simulink library "DQN_Lib (conflicted copy 2023-11-25 155310)"  (R2023b)
settings: Solver=VariableStepAuto  StartTime=0.0  StopTime=10.0  RelTol=1e-3
undefined symbols (not defined in the file): FreqRad, HrmOrd, Init, La, N, R, Ra, TimeStep, Ts, Ts_dqn, Ws
libraries: $bdroot x4, spsMeanVariableFrequencyLib x4, eeTransforms x3, spsabctodq0Lib x2, spsAlphaBetaZerotodq0Lib x1
(part 5 of 8)

== matlab function DQN_Lib (conflicted copy 2023-11-25 155310)/DQn->ABC11 ==
  data: Xdc input size=3; Xdp input; Xdn input; Xdz input; Xqp input; Xqn input; Xqz input; th input; abc output; N parameter
%function abc = Mult(Z0,Zdp,Zqp,Zdn,Zqn,Zdz,Zqz,th, N)
function abc = dqn2abc(Xdc,Xdp,Xdn,Xdz,Xqp,Xqn,Xqz,th,N)



abc   = [Xdc(1);Xdc(2);Xdc(3)];
abc3p = [0;0;0];
abc3n = [0;0;0];
abc1p = [0;0;0];
%abc1n = [0;0;0];
   

for i = 1 : N
    abc3p = abc3p + [sin(i*th)*Xdp(i)           + cos(i*th)*Xqp(i);
                     sin(i*th-2*pi/3)*Xdp(i)    + cos(i*th-2*pi/3)*Xqp(i);
                     sin(i*th+2*pi/3)*Xdp(i)    + cos(i*th+2*pi/3)*Xqp(i)];
                 
    abc3n = abc3n + [sin(-i*th)*Xdn(i)          + cos(-i*th)*Xqn(i);
                     sin(-i*th-2*pi/3)*Xdn(i)   + cos(-i*th-2*pi/3)*Xqn(i);
                     sin(-i*th+2*pi/3)*Xdn(i)   + cos(-i*th+2*pi/3)*Xqn(i)];
                 
    abc1p = abc1p + [sin(i*th)*Xdz(i)           + cos(i*th)*Xqz(i);
                     sin(i*th-0*2*pi/3)*Xdz(i)  + cos(i*th-0*2*pi/3)*Xqz(i);
                     sin(i*th+0*2*pi/3)*Xdz(i)  + cos(i*th+0*2*pi/3)*Xqz(i)];  
 
%     abc1n = abc1n + [sin(-i*th)*D1n(i)           + cos(-i*th)*Q1n(i);
%                      sin(-i*th-0*2*pi/3)*D1n(i)  + cos(-i*th-0*2*pi/3)*Q1n(i);
%                      sin(-i*th+0*2*pi/3)*D1n(i)  + cos(-i*th+0*2*pi/3)*Q1n(i)];  
                 
end

abc = abc+abc3p+abc3n+abc1p;%+abc1n;

== matlab function DQN_Lib (conflicted copy 2023-11-25 155310)/MATLAB Function ==
  data: Xdp input; X_DQN output; Xdn input; Xdz input; Xqp input; Xqn input; Xqz input; N parameter
function X_DQN = fcn(Xdp, Xdn, Xdz, Xqp, Xqn, Xqz, N)

    X_DQN = zeros(N+1,6);

    X_DQN(:,1) = Xdp;
    X_DQN(:,2) = Xdn;
    X_DQN(:,3) = Xdz;
    X_DQN(:,4) = Xqp;
    X_DQN(:,5) = Xqn;
    X_DQN(:,6) = Xqz;

end

== matlab function DQN_Lib (conflicted copy 2023-11-25 155310)/Int_DQN_fdbk/Int_d_2N_2 ==
  settings: updateMethod=DISCRETE
  data: Zdp output; Xdp input; Xdn input; Xdz input; Xqp input; Xqn input; Xqz input; Zdn output; N parameter; dt parameter; w parameter; Zdz output; Zqp output; Zqn output; Zqz output; R parameter; iL parameter; SW parameter
function [Zdp,Zdn,Zdz,Zqp,Zqn,Zqz]  = IntDQN(Xdp, Xdn, Xdz, Xqp, Xqn, Xqz, N, dt, w, R, iL, SW)

    persistent Zdc_old;    
    persistent Xdc_old;   
    persistent Zdp_old;    
    persistent Zqp_old;    
    persistent Zdn_old;    
    persistent Zqn_old;    
    persistent Zdz_old;    
    persistent Zqz_old;  
    persistent Krl1;
    persistent Krl2;
       
    persistent dt2;
    persistent range;
       
    Xdc = zeros(6,1);
    Zdc = zeros(6,1);
    
    Xdc(1) = Xdp(1);
    Xdc(2) = Xdn(1);
    Xdc(3) = Xdz(1);
    Xdc(4) = Xqp(1);
    Xdc(5) = Xqn(1);
    Xdc(6) = Xqz(1);

    Xdp = [Xdp(2:end); zeros(N-numel(Xdp)+1,1)];
    Xqp = [Xqp(2:end); zeros(N-numel(Xqp)+1,1)];
    Xdn = [Xdn(2:end); zeros(N-numel(Xdn)+1,1)];
    Xqn = [Xqn(2:end); zeros(N-numel(Xqn)+1,1)];
    Xdz = [Xdz(2:end); zeros(N-numel(Xdz)+1,1)];
    Xqz = [Xqz(2:end); zeros(N-numel(Xqz)+1,1)];
       
    Zdp = zeros(N+1,1);
    Zdn = zeros(N+1,1);
    Zqp = zeros(N+1,1);
    Zqn = zeros(N+1,1);
    Zdz = zeros(N+1,1);
    Zqz = zeros(N+1,1);
       
    if(isempty(Zdp_old)) 
        Zdc_old  = zeros(6,1); %Zdc_old  = InitInt';
        Xdc_old  = zeros(6,1);
        
        Zdp_old  = zeros(N,1);% Zdp_old(1) = InitInt(1);
        Zdn_old  = zeros(N,1);% Zdn_old(1) = InitInt(2);
        Zdz_old  = zeros(N,1);% Zdz_old(1) = InitInt(3);
        Zqp_old  = zeros(N,1);% Zqp_old(1) = InitInt(4);
        Zqn_old  = zeros(N,1);% Zqn_old(1) = InitInt(5);
        Zqz_old  = zeros(N,1);% Zqz_old(1) = InitInt(6);
        
        dt2 = dt/2;  
        range = N; 
        
        if(SW)
            Krl1 = (iL/(1+dt2*R*iL));
            Krl2 = (1-dt2*R*iL)/(1+dt2*R*iL);
        else
            Krl1 = 1;
            Krl2 = 1;
        end
        
    end

    
    
    %Zdc(:) = dt2*(Xdc(:)+Xdc_old(:))+Zdc_old(:);
    Zdc(:) = Krl1*dt2*(Xdc(:)+Xdc_old(:))+Krl2*Zdc_old(:);
    
    
    Zdc_old = Zdc;
    Xdc_old = Xdc;
    
    if(N>0)
              
        for i = 1 : range

            wn =  i * w;
            wndt2 = wn*dt2;
            A = 2*dt2/(1+wndt2^2);
            B = (1-wndt2^2)/(1+wndt2^2);

            %%% NEG %%%
            Zdp(i) = Krl1*A*(Xdp(i)+wndt2*Xqp(i))+Krl2*(B*Zdp_old(i)+A*wn*Zqp_old(i));
            Zqp(i) = Krl1*A*(Xqp(i)-wndt2*Xdp(i))+Krl2*(B*Zqp_old(i)-A*wn*Zdp_old(i));

            Zdp_old(i) = Zdp(i);
            Zqp_old(i) = Zqp(i); 


            %%% NEG %%%
            Zdn(i) = Krl1*A*(Xdn(i)-wndt2*Xqn(i))+Krl2*(B*Zdn_old(i)-A*wn*Zqn_old(i));
            Zqn(i) = Krl1*A*(Xqn(i)+wndt2*Xdn(i))+Krl2*(B*Zqn_old(i)+A*wn*Zdn_old(i));

            Zdn_old(i) = Zdn(i);
            Zqn_old(i) = Zqn(i); 

            %%% ZERO %%%
            Zdz(i) = Krl1*A*(Xdz(i)+wndt2*Xqz(i))+Krl2*(B*Zdz_old(i)+A*wn*Zqz_old(i));
            Zqz(i) = Krl1*A*(Xqz(i)-wndt2*Xdz(i))+Krl2*(B*Zqz_old(i)-A*wn*Zdz_old(i));

            Zdz_old(i) = Zdz(i);
            Zqz_old(i) = Zqz(i); 
        end

        Zdp(2:end) = Zdp(1:end-1);
        Zdn(2:end) = Zdn(1:end-1);
        Zdz(2:end) = Zdz(1:end-1);
        Zqp(2:end) = Zqp(1:end-1);
        Zqn(2:end) = Zqn(1:end-1);
        Zqz(2:end) = Zqz(1:end-1);


    end
    
    Zdp(1)     = Zdc(1);
    Zdn(1)     = Zdc(2);
    Zdz(1)     = Zdc(3);
    Zqp(1)     = Zdc(4);
    Zqn(1)     = Zdc(5);
    Zqz(1)     = Zdc(6);
end

== matlab function DQN_Lib (conflicted copy 2023-11-25 155310)/MatMultDQN ==
  settings: updateMethod=DISCRETE
  data: X_DQN input; Y_DQN output; R parameter; H parameter; chkInv parameter
function Y_DQN  = MatMultDQN(X_DQN, R, H, chkInv)
    persistent Rd_DQN;
    persistent Rdc;

    %%%%%%%%%%%%%%%%%%%%%%%%%%%%%%%%%%%%%%%%%
    %
    %  X_DQN.rows: H+1 (N+1); X_DQN.cols: 6*nrSignals
    %  
    %  R.rows: NN ; R.cols: X_DQN.cols; Rows and cols must be div. by 3
    %
    %  Y_DQN: rows_size: H+1 (N+1); cols_size: 6xR.rows
    %
    %%%%%%%%%%%%%%%%%%%%%%%%%%%%%%%%%%%%%%%%%%
    
    if(mod(size(R,1),3) ~= 0 || mod(size(R,2),3) ~= 0)
        error('[RD] The input matrix is in the wrong form!');
    end
    
    mrows = size(R,1)/3; %signal size
    mcols = size(R,2)/3; %signal size
    
    Y_DQN = zeros(1*H+1,6*mrows);

    if(isempty(Rd_DQN))
        
        Rd_DQN = zeros(6*mrows,6*mcols);
        Rdc = zeros(6*(mrows),6*mcols);
        a = -0.5+0.866i;
        a2 = -0.5-0.866i;
        S = [1,a,a2;1,a2,a;1,1,1]/3;
        
        for i = 1 : mrows
            for j = 1 : mcols
                oi = (i-1)*6;
                oj = (j-1)*6;
                A_120 = S*R((1:3) + (i-1)*3,(1:3) + (j-1)*3)/S;

                Rd_DQN(oi+1,oj+1) =  real(A_120(1,1)); Rd_DQN(oi+1,oj+2) = -real(A_120(1,2)); Rd_DQN(oi+1,oj+3) =  real(A_120(1,3)); 
                Rd_DQN(oi+1,oj+4) = -imag(A_120(1,1)); Rd_DQN(oi+1,oj+5) = -imag(A_120(1,2)); Rd_DQN(oi+1,oj+6) = -imag(A_120(1,3));
                Rd_DQN(oi+2,oj+1) = -real(A_120(2,1)); Rd_DQN(oi+2,oj+2) =  real(A_120(2,2)); Rd_DQN(oi+2,oj+3) = -real(A_120(2,3)); 
                Rd_DQN(oi+2,oj+4) =  imag(A_120(2,1)); Rd_DQN(oi+2,oj+5) =  imag(A_120(2,2)); Rd_DQN(oi+2,oj+6) =  imag(A_120(2,3));
                Rd_DQN(oi+3,oj+1) =  real(A_120(3,1)); Rd_DQN(oi+3,oj+2) = -real(A_120(3,2)); Rd_DQN(oi+3,oj+3) =  real(A_120(3,3)); 
                Rd_DQN(oi+3,oj+4) = -imag(A_120(3,1)); Rd_DQN(oi+3,oj+5) = -imag(A_120(3,2)); Rd_DQN(oi+3,oj+6) = -imag(A_120(3,3));

                Rd_DQN(oi+4,oj+1) =  imag(A_120(1,1)); Rd_DQN(oi+4,oj+2) = -imag(A_120(1,2)); Rd_DQN(oi+4,oj+3) =  imag(A_120(1,3)); 
                Rd_DQN(oi+4,oj+4) =  real(A_120(1,1)); Rd_DQN(oi+4,oj+5) =  real(A_120(1,2)); Rd_DQN(oi+4,oj+6) =  real(A_120(1,3));
                Rd_DQN(oi+5,oj+1) =  imag(A_120(2,1)); Rd_DQN(oi+5,oj+2) = -imag(A_120(2,2)); Rd_DQN(oi+5,oj+3) =  imag(A_120(2,3)); 
                Rd_DQN(oi+5,oj+4) =  real(A_120(2,1)); Rd_DQN(oi+5,oj+5) =  real(A_120(2,2)); Rd_DQN(oi+5,oj+6) =  real(A_120(2,3));
                Rd_DQN(oi+6,oj+1) =  imag(A_120(3,1)); Rd_DQN(oi+6,oj+2) = -imag(A_120(3,2)); Rd_DQN(oi+6,oj+3) =  imag(A_120(3,3)); 
                Rd_DQN(oi+6,oj+4) =  real(A_120(3,1)); Rd_DQN(oi+6,oj+5) =  real(A_120(3,2)); Rd_DQN(oi+6,oj+6) =  real(A_120(3,3));

                Tad_p = [0      -sqrt(1/3)   sqrt(1/3);
                        (2/3)   -(1/3)      -(1/3);
                        (1/3)    (1/3)       (1/3)];

                Tda_p = [-0           1     1;
                         -sqrt(3/4)  -0.5   1;
                          sqrt(3/4)  -0.5   1;];

                Tdqn_a = [Tda_p(:,1)  Tda_p(:,1)  0*Tda_p(:,3)  Tda_p(:,2)  Tda_p(:,2)  2*Tda_p(:,3)]/2;
                Ta_dqn = [Tad_p(1,:); Tad_p(1,:); 0*Tad_p(3,:); Tad_p(2,:); Tad_p(2,:); Tad_p(3,:)];

                if(chkInv)
                    Rd_DQN = eye(6)/Rd_DQN;
                    Rdc(oi+1:oi+6,:) = (Ta_dqn*(eye(3)/R((1:3) + (i-1)*3,(1:3) + (j-1)*3))*Tdqn_a);
                else
                    Rdc(oi+1:oi+6,oj+1:oj+6) = (Ta_dqn*R((1:3) + (i-1)*3,(1:3) + (j-1)*3)*Tdqn_a);
                end
        
            end
        end
        
    end

    for i = 1 : mrows
        for j = 1 : mcols
            oi = (i-1)*6;
            oj = (j-1)*6;
            %Y_DQN(1,oi+1:oi+6) = (Rdc(oi+1:oi+6,:)*X_DQN(1,:)')';
            Y_DQN(1,oi+1:oi+6) = X_DQN(1,:)*Rdc(oi+1:oi+6,:)';
            if(H>0)
                %Y_DQN(2:end,oi+1:oi+6) = Y_DQN(2:end,oi+1:oi+6) + (Rd_DQN(oi+1:oi+6,oj+1:oj+6)*X_DQN(2:end,oj+1:oj+6)')';
                Y_DQN(2:end,oi+1:oi+6) = Y_DQN(2:end,oi+1:oi+6) + X_DQN(2:end,oj+1:oj+6)*Rd_DQN(oi+1:oi+6,oj+1:oj+6);
            end
        end
    end
end

== matlab function DQN_Lib (conflicted copy 2023-11-25 155310)/MATLAB Function3 ==
  data: Xdc input size=3; dZdc output size=3; Xdp input; Xdn input; Xdz input; Xqp input; Xqn input; Xqz input; dZdp output; dZdn output; dZdz output; dZqp output; dZqn output; dZqz output; N parameter; w parameter; EMT parameter; Ts parameter
function [dZdc,dZdp,dZdn,dZdz,dZqp,dZqn,dZqz]  = DerDQN(Xdc, Xdp, Xdn, Xdz, Xqp, Xqn, Xqz, N, w, EMT, Ts)

    dZdc = zeros(3,1);
    
    
    persistent Xdp_old;
    persistent Xqp_old;
    persistent Xdn_old;
    persistent Xqn_old;
    persistent Xdz_old;
    persistent Xqz_old;
    if(isempty(Xdp_old))  Xdp_old     = zeros(N,1); end
    if(isempty(Xqp_old))  Xqp_old     = zeros(N,1); end
    if(isempty(Xdn_old))  Xdn_old     = zeros(N,1); end
    if(isempty(Xqn_old))  Xqn_old     = zeros(N,1); end    
    if(isempty(Xdz_old))  Xdz_old     = zeros(N,1); end
    if(isempty(Xqz_old))  Xqz_old     = zeros(N,1); end    
    

    Xdp = [Xdp; zeros(N-numel(Xdp),1)];
    Xqp = [Xqp; zeros(N-numel(Xqp),1)];
      
    Xdn = [Xdn; zeros(N-numel(Xdn),1)];
    Xqn = [Xqn; zeros(N-numel(Xqn),1)];
    
    Xdz = [Xdz; zeros(N-numel(Xdz),1)];
    Xqz = [Xqz; zeros(N-numel(Xqz),1)];
       
    dZdp = zeros(N,1);
    dZdn = zeros(N,1);
    dZqp = zeros(N,1);
    dZqn = zeros(N,1);
    dZdz = zeros(N,1);
    dZqz = zeros(N,1);
    
    
    for i = 1 : N
        wn = i*w;
        if(EMT)
            dZdp(i) = (Xdp(i)-Xdp_old(i))/Ts;
            Xdp_old(i) = Xdp(i);
            
            dZqp(i) = (Xqp(i)-Xqp_old(i))/Ts;
            Xqp_old(i) = Xqp(i);
            
            dZdn(i) = (Xdn(i)-Xdn_old(i))/Ts;
            Xdn_old(i) = Xdn(i);
            
            dZqn(i) = (Xqn(i)-Xqn_old(i))/Ts;
            Xqn_old(i) = Xqn(i);
            
            dZdz(i) = (Xdz(i)-Xdz_old(i))/Ts;
            Xdz_old(i) = Xdz(i);
            
            dZqz(i) = (Xqz(i)-Xqz_old(i))/Ts;
            Xqz_old(i) = Xqz(i);
        end
        
        dZdp(i) = dZdp(i) + Xqp(i)*(-(wn));
        dZqp(i) = dZqp(i) + Xdp(i)*((wn)); 

        dZdn(i) = dZdn(i) + Xqn(i)*((wn));
        dZqn(i) = dZqn(i) + Xdn(i)*(-(wn)); 

        dZdz(i) = dZdz(i) + Xqz(i)*(-(wn));
        dZqz(i) = dZqz(i) + Xdz(i)*((wn)); 
    end

end

== matlab function DQN_Lib (conflicted copy 2023-11-25 155310)/VecMultDQN ==
  data: X_DQN input; Y_DQN output; R parameter; H parameter; chkInv parameter
function Y_DQN  = MatMultDQN(X_DQN, R, H, chkInv)
    persistent Rd_DQN;
    persistent Rdc;
    
    if(size(R,1) ~= 3 || size(R,2) ~= 3)
        error('The input matrix needs to be 3x3!');
    end
    
    Z_DQN = zeros(1*H+1,6);
    X_DQN = reshape(X_DQN,[],6);
    Y_DQN = zeros((1*H+1)*6,1);

    if(isempty(Rd_DQN))
        
        Rd_DQN = zeros(6,6);
        a = -0.5+0.866i;
        a2 = -0.5-0.866i;
        S = [1,a,a2;1,a2,a;1,1,1]/3;
        A_120 = S*R/S;

        Rd_DQN(1,1) =  real(A_120(1,1)); Rd_DQN(1,2) = -real(A_120(1,2)); Rd_DQN(1,3) =  real(A_120(1,3)); 
        Rd_DQN(1,4) = -imag(A_120(1,1)); Rd_DQN(1,5) = -imag(A_120(1,2)); Rd_DQN(1,6) = -imag(A_120(1,3));
        Rd_DQN(2,1) = -real(A_120(2,1)); Rd_DQN(2,2) =  real(A_120(2,2)); Rd_DQN(2,3) = -real(A_120(2,3)); 
        Rd_DQN(2,4) =  imag(A_120(2,1)); Rd_DQN(2,5) =  imag(A_120(2,2)); Rd_DQN(2,6) =  imag(A_120(2,3));
        Rd_DQN(3,1) =  real(A_120(3,1)); Rd_DQN(3,2) = -real(A_120(3,2)); Rd_DQN(3,3) =  real(A_120(3,3)); 
        Rd_DQN(3,4) = -imag(A_120(3,1)); Rd_DQN(3,5) = -imag(A_120(3,2)); Rd_DQN(3,6) = -imag(A_120(3,3));

        Rd_DQN(4,1) =  imag(A_120(1,1)); Rd_DQN(4,2) = -imag(A_120(1,2)); Rd_DQN(4,3) =  imag(A_120(1,3)); 
        Rd_DQN(4,4) =  real(A_120(1,1)); Rd_DQN(4,5) =  real(A_120(1,2)); Rd_DQN(4,6) =  real(A_120(1,3));
        Rd_DQN(5,1) =  imag(A_120(2,1)); Rd_DQN(5,2) = -imag(A_120(2,2)); Rd_DQN(5,3) =  imag(A_120(2,3)); 
        Rd_DQN(5,4) =  real(A_120(2,1)); Rd_DQN(5,5) =  real(A_120(2,2)); Rd_DQN(5,6) =  real(A_120(2,3));
        Rd_DQN(6,1) =  imag(A_120(3,1)); Rd_DQN(6,2) = -imag(A_120(3,2)); Rd_DQN(6,3) =  imag(A_120(3,3)); 
        Rd_DQN(6,4) =  real(A_120(3,1)); Rd_DQN(6,5) =  real(A_120(3,2)); Rd_DQN(6,6) =  real(A_120(3,3));

        Tad_p = [0      -sqrt(1/3)   sqrt(1/3);
                (2/3)   -(1/3)      -(1/3);
                (1/3)    (1/3)       (1/3)];

        Tda_p = [-0           1     1;
                 -sqrt(3/4)  -0.5   1;
                  sqrt(3/4)  -0.5   1;];
             
        Tdqn_a = [Tda_p(:,1)  Tda_p(:,1)  0*Tda_p(:,3)  Tda_p(:,2)  Tda_p(:,2)  2*Tda_p(:,3)]/2;
        Ta_dqn = [Tad_p(1,:); Tad_p(1,:); 0*Tad_p(3,:); Tad_p(2,:); Tad_p(2,:); Tad_p(3,:)];
        
        if(chkInv)
            Rd_DQN = eye(6)/Rd_DQN;
            Rdc = (Ta_dqn*(eye(3)/R)*Tdqn_a);
        else
            Rdc = (Ta_dqn*R*Tdqn_a);
        end
    end

    Z_DQN(1,:)     = (Rdc*X_DQN(1,:)')';
    if(H>0)
        Z_DQN(2:end,:) = (Rd_DQN*X_DQN(2:end,:)')';
    end
    Y_DQN = reshape(Z_DQN,6*(H+1),1);

end

== matlab function DQN_Lib (conflicted copy 2023-11-25 155310)/BACKUP/MatMultDQN1 ==
  data: X_DQN input; Y_DQN output; R parameter; H parameter; chkInv parameter
function Y_DQN  = MatMultDQN(X_DQN, R, H, chkInv)
    persistent Rd_DQN;
    persistent Rdc;
    
    if(mod(size(R,1),3) ~= 0 || size(R,2) ~= 3)
        error('The input matrix needs to be Nx3!');
    end
    
    Y_DQN = zeros(1*H+1,6);

    if(isempty(Rd_DQN))
        
        Rd_DQN = zeros(6*(size(R,1)/3),6);
        a = -0.5+0.866i;
        a2 = -0.5-0.866i;
        S = [1,a,a2;1,a2,a;1,1,1]/3;
        A_120 = S*R/S;

        Rd_DQN(1,1) =  real(A_120(1,1)); Rd_DQN(1,2) = -real(A_120(1,2)); Rd_DQN(1,3) =  real(A_120(1,3)); 
        Rd_DQN(1,4) = -imag(A_120(1,1)); Rd_DQN(1,5) = -imag(A_120(1,2)); Rd_DQN(1,6) = -imag(A_120(1,3));
        Rd_DQN(2,1) = -real(A_120(2,1)); Rd_DQN(2,2) =  real(A_120(2,2)); Rd_DQN(2,3) = -real(A_120(2,3)); 
        Rd_DQN(2,4) =  imag(A_120(2,1)); Rd_DQN(2,5) =  imag(A_120(2,2)); Rd_DQN(2,6) =  imag(A_120(2,3));
        Rd_DQN(3,1) =  real(A_120(3,1)); Rd_DQN(3,2) = -real(A_120(3,2)); Rd_DQN(3,3) =  real(A_120(3,3)); 
        Rd_DQN(3,4) = -imag(A_120(3,1)); Rd_DQN(3,5) = -imag(A_120(3,2)); Rd_DQN(3,6) = -imag(A_120(3,3));

        Rd_DQN(4,1) =  imag(A_120(1,1)); Rd_DQN(4,2) = -imag(A_120(1,2)); Rd_DQN(4,3) =  imag(A_120(1,3)); 
        Rd_DQN(4,4) =  real(A_120(1,1)); Rd_DQN(4,5) =  real(A_120(1,2)); Rd_DQN(4,6) =  real(A_120(1,3));
        Rd_DQN(5,1) =  imag(A_120(2,1)); Rd_DQN(5,2) = -imag(A_120(2,2)); Rd_DQN(5,3) =  imag(A_120(2,3)); 
        Rd_DQN(5,4) =  real(A_120(2,1)); Rd_DQN(5,5) =  real(A_120(2,2)); Rd_DQN(5,6) =  real(A_120(2,3));
        Rd_DQN(6,1) =  imag(A_120(3,1)); Rd_DQN(6,2) = -imag(A_120(3,2)); Rd_DQN(6,3) =  imag(A_120(3,3)); 
        Rd_DQN(6,4) =  real(A_120(3,1)); Rd_DQN(6,5) =  real(A_120(3,2)); Rd_DQN(6,6) =  real(A_120(3,3));

        Tad_p = [0      -sqrt(1/3)   sqrt(1/3);
                (2/3)   -(1/3)      -(1/3);
                (1/3)    (1/3)       (1/3)];

        Tda_p = [-0           1     1;
                 -sqrt(3/4)  -0.5   1;
                  sqrt(3/4)  -0.5   1;];
             
        Tdqn_a = [Tda_p(:,1)  Tda_p(:,1)  0*Tda_p(:,3)  Tda_p(:,2)  Tda_p(:,2)  2*Tda_p(:,3)]/2;
        Ta_dqn = [Tad_p(1,:); Tad_p(1,:); 0*Tad_p(3,:); Tad_p(2,:); Tad_p(2,:); Tad_p(3,:)];
        
        if(chkInv)
            Rd_DQN = eye(6)/Rd_DQN;
            Rdc = (Ta_dqn*(eye(3)/R)*Tdqn_a);
        else
            Rdc = (Ta_dqn*R*Tdqn_a);
        end
    end

    Y_DQN(1,:)     = (Rdc*X_DQN(1,:)')';
    if(H>0)
        Y_DQN(2:end,:) = (Rd_DQN*X_DQN(2:end,:)')';
    end
end

== matlab function DQN_Lib (conflicted copy 2023-11-25 155310)/BACKUP/Int_DQN_Mat ==
  settings: updateMethod=DISCRETE
  data: Z_DQN output; X_DQN input; N parameter; dt parameter; w parameter; EMT parameter; InitInt parameter
function Z_DQN   = Int_DQN_Mat(X_DQN, N, dt, w, EMT, InitInt)

    persistent Zdc_old;    
    persistent Xdc_old;   
    persistent Zdp_old;    
    persistent Zqp_old;    
    persistent Zdn_old;    
    persistent Zqn_old;    
    persistent Zdz_old;    
    persistent Zqz_old;  
    
    persistent Xdp_old;    
    persistent Xqp_old;    
    persistent Xdn_old;    
    persistent Xqn_old;    
    persistent Xdz_old;    
    persistent Xqz_old;
    
    Xdp = X_DQN(:,1);
    Xdn = X_DQN(:,2);
    Xdz = X_DQN(:,3);
    Xqp = X_DQN(:,4);
    Xqn = X_DQN(:,5);
    Xqz = X_DQN(:,6);
    
    Z_DQN = zeros(1*N+1,6);
    
    dt2 = dt/2;

    Tad_p2 = (2/3)*[sin(0) sin(0-2*pi/3) sin(0+2*pi/3);  
                   cos(0) cos(0-2*pi/3) cos(0+2*pi/3);];

    Tad_z2 = (1/3)*[sin(0) sin(0) sin(0);  
                   cos(0) cos(0) cos(0);];

    Ta_dqn = [Tad_p2(1,:); Tad_p2(1,:); Tad_z2(1,:); Tad_p2(2,:); Tad_p2(2,:); Tad_z2(2,:)];
    
    Xdc = zeros(6,1);
    Zdc = zeros(6,1);
    
    Xdc(1) = Xdp(1);
    Xdc(2) = Xdn(1);
    Xdc(3) = Xdz(1);
    Xdc(4) = Xqp(1);
    Xdc(5) = Xqn(1);
    Xdc(6) = Xqz(1);

    Xdp = [Xdp(2:end); zeros(N-numel(Xdp)+1,1)];
    Xqp = [Xqp(2:end); zeros(N-numel(Xqp)+1,1)];
    Xdn = [Xdn(2:end); zeros(N-numel(Xdn)+1,1)];
    Xqn = [Xqn(2:end); zeros(N-numel(Xqn)+1,1)];
    Xdz = [Xdz(2:end); zeros(N-numel(Xdz)+1,1)];
    Xqz = [Xqz(2:end); zeros(N-numel(Xqz)+1,1)];
       
    Zdp = zeros(N+1,1);
    Zdn = zeros(N+1,1);
    Zqp = zeros(N+1,1);
    Zqn = zeros(N+1,1);
    Zdz = zeros(N+1,1);
    Zqz = zeros(N+1,1);
    
    if(isempty(Zdc_old)) Zdc_old  = InitInt';   end
    if(isempty(Xdc_old)) Xdc_old  = zeros(6,1); end
    
    Zdc(:) = dt2*(Xdc(:)+Xdc_old(:))+Zdc_old(:);
    Zdc_old = Zdc;
    Xdc_old = Xdc;


    if(N>0)

        if(1)
            if(isempty(Zdp_old)) Zdp_old  = zeros(N,1); end
            if(isempty(Zqp_old)) Zqp_old  = zeros(N,1); end     
            if(isempty(Zdn_old)) Zdn_old  = zeros(N,1); end
            if(isempty(Zqn_old)) Zqn_old  = zeros(N,1); end
            if(isempty(Zdz_old)) Zdz_old  = zeros(N,1); end
            if(isempty(Zqz_old)) Zqz_old  = zeros(N,1); end
        else
            
            if(isempty(Zdp_old)) Zdp_old  = zeros(N,1); Zdp_old(1) = InitInt(1); end
            if(isempty(Zdn_old)) Zdn_old  = zeros(N,1); Zdn_old(1) = InitInt(2); end
            if(isempty(Zdz_old)) Zdz_old  = zeros(N,1); Zdz_old(1) = InitInt(3); end
            if(isempty(Zqp_old)) Zqp_old  = zeros(N,1); Zqp_old(1) = InitInt(4); end 
            if(isempty(Zqn_old)) Zqn_old  = zeros(N,1); Zqn_old(1) = InitInt(5); end
            if(isempty(Zqz_old)) Zqz_old  = zeros(N,1); Zqz_old(1) = InitInt(6); end
        end
        
        if(isempty(Xdp_old)) Xdp_old  = zeros(N,1); end
        if(isempty(Xqp_old)) Xqp_old  = zeros(N,1); end
        if(isempty(Xdn_old)) Xdn_old  = zeros(N,1); end
        if(isempty(Xqn_old)) Xqn_old  = zeros(N,1); end
        if(isempty(Xdz_old)) Xdz_old  = zeros(N,1); end
        if(isempty(Xqz_old)) Xqz_old  = zeros(N,1); end

        %A = zeros(1,N);
        A = 0;

        for i = 1 : N
            wn =  i * w; 

            if(EMT)

%                 if(~isempty(A(i)))
%                     A(i) = 2/(1+(dt2*wn)^2);
%                 end
                A = 2/(1+(dt2*wn)^2);

                wndt2 = wn*dt2;

                %%% POS %%%
                K1 = dt2*(2*Xdp(i)+Zqp_old(i)*wn) + Zdp_old(i);
                K2 = dt2*(2*Xqp(i)-Zdp_old(i)*wn) + Zqp_old(i);

                Zdp(i) = A*( K1 + wndt2*K2)/2;
                Zqp(i) = A*( K2 - wndt2*K1)/2;

                Zdp_old(i) = Zdp(i);
                Zqp_old(i) = Zqp(i); 

                %%% NEG %%%
                K1 = dt2*(2*Xdn(i)-Zqn_old(i)*wn) + Zdn_old(i);
                K2 = dt2*(2*Xqn(i)+Zdn_old(i)*wn) + Zqn_old(i);

                Zdn(i) = A*( K1 - wndt2*K2)/2;
                Zqn(i) = A*( K2 + wndt2*K1)/2;

                Zdn_old(i) = Zdn(i);
                Zqn_old(i) = Zqn(i);

                %%% ZERO %%%
                K1 = dt2*(2*Xdz(i)+Zqz_old(i)*wn) + Zdz_old(i);
                K2 = dt2*(2*Xqz(i)-Zdz_old(i)*wn) + Zqz_old(i);

                Zdz(i) = A*( K1 + wndt2*K2)/2;
                Zqz(i) = A*( K2 - wndt2*K1)/2;

                Zdz_old(i) = Zdz(i);
                Zqz_old(i) = Zqz(i);

            else

                Zdp(i) = (Xqp(i))*(1/(wn));
                Zqp(i) = (Xdp(i))*(-1/(wn)); 

                Zdn(i) = (Xqn(i))*(-1/(wn));
                Zqn(i) = (Xdn(i))*(1/(wn)); 

                Zdz(i) = (Xqz(i))*(1/(wn));
                Zqz(i) = (Xdz(i))*(-1/(wn));

                sT = sin(2*pi/3);
                cT = cos(2*pi/3);

                Zdc = Zdc-Ta_dqn*[Zqp(i);-sT*Zdp(i)+cT*Zqp(i);sT*Zdp(i)+cT*Zqp(i)];
                Zdc = Zdc-Ta_dqn*[Zqn(i);-sT*Zdn(i)+cT*Zqn(i);sT*Zdn(i)+cT*Zqn(i)];
                Zdc = Zdc-Ta_dqn*[Zqz(i); Zqz(i)             ;Zqz(i)];

            end
            

        end

        Zdp(2:end) = Zdp(1:end-1);
        Zdn(2:end) = Zdn(1:end-1);
        Zdz(2:end) = Zdz(1:end-1);
        Zqp(2:end) = Zqp(1:end-1);
        Zqn(2:end) = Zqn(1:end-1);
        Zqz(2:end) = Zqz(1:end-1);


    end

    Zdp(1)     = Zdc(1);
    Zdn(1)     = Zdc(2);
    Zdz(1)     = Zdc(3);
    Zqp(1)     = Zdc(4);
    Zqn(1)     = Zdc(5);
    Zqz(1)     = Zdc(6);
    
    
    Z_DQN(:,1) = Zdp;
    Z_DQN(:,2) = Zdn;
    Z_DQN(:,3) = Zdz;
    Z_DQN(:,4) = Zqp;
    Z_DQN(:,5) = Zqn;
    Z_DQN(:,6) = Zqz;
end

== matlab function DQN_Lib (conflicted copy 2023-11-25 155310)/MATLAB Function4 ==
  data: Xdcpnz_c input; Y_DQN output
function Y_DQN  = f012C2DQN(Xdcpnz_c)

    if(size(Xdcpnz_c,2) < 2)
        error('Wrong size!');
    end
    
    N = size(Xdcpnz_c,2)-1;
    Y_DQN = zeros(N+1,6);

    Y_DQN(1,4) =  2*real(Xdcpnz_c(1,1));
    Y_DQN(1,5) =  2*real(Xdcpnz_c(2,1));
    Y_DQN(1,6) =  real(Xdcpnz_c(3,1));

    Y_DQN(1,1) =  -2*imag(Xdcpnz_c(1,1));
    Y_DQN(1,2) =  2*imag(Xdcpnz_c(2,1));
    Y_DQN(1,3) =  imag(Xdcpnz_c(3,1));
    
    for i = 2 : N + 1
    
        Y_DQN(i,1) =  real(Xdcpnz_c(1,i));
        Y_DQN(i,2) = -real(Xdcpnz_c(2,i));
        Y_DQN(i,3) =  real(Xdcpnz_c(3,i));

        Y_DQN(i,4) =  imag(Xdcpnz_c(1,i));
        Y_DQN(i,5) =  imag(Xdcpnz_c(2,i));
        Y_DQN(i,6) =  imag(Xdcpnz_c(3,i));
    
    end


end

== matlab function DQN_Lib (conflicted copy 2023-11-25 155310)/Mult_DQNc_Mat ==
  data: Xdcpnz_c input; Ydcpnz_c input; N parameter; HrmDbl parameter; Zdcpnz_c output
function Zdcpnz_c    = fMultDQNc(Xdcpnz_c, Ydcpnz_c, N, HrmDbl)
    Zdcpnz_c = complex(zeros(3,2*N+1));

    persistent T132;
    persistent T213;
    persistent T231;
    persistent T321;
    persistent T312;
    persistent Sas;
    persistent Ssa;

    if(isempty(T132)) 
        T132 = [1 0 0; 0 0 1; 0 1 0];
        T213 = [0 1 0; 1 0 0; 0 0 1];
        T231 = [0 1 0; 0 0 1; 1 0 0];
        T321 = [0 0 1; 0 1 0; 1 0 0];
        T312 = [0 0 1; 1 0 0; 0 1 0];

        a = -0.5+0.866i;
        a2 = -0.5-0.866i;
        Sas = [1,a,a2;1,a2,a;1,1,1]/3;
        Ssa = eye(3)/(Sas);
    end

%%%%%%%%%%%%%%%%%%%%%%%%%%%%%%

    Zdcpnz_c(:,1) = Sas*(Ssa*Xdcpnz_c(:,1).*Ssa*Ydcpnz_c(:,1));

    sX = size(Xdcpnz_c,2);
    Xdcpnz_c = [Xdcpnz_c zeros(3,N+1-sX)];

    sY = size(Ydcpnz_c,2);
    Ydcpnz_c = [Ydcpnz_c zeros(3,N+1-sY)];

       
    for h = 1 : 2*N
        if(h<=N)

            Zdcpnz_c(3,1) = Zdcpnz_c(3,1) + 0.5*real(Xdcpnz_c(:,h+1)'*Ydcpnz_c(:,h+1));


            Zdcpnz_c(3,2*h+1) = Zdcpnz_c(3,2*h+1) + 0.5*Xdcpnz_c(1,h+1)*Ydcpnz_c(2,h+1)*exp(-1i*pi/2);

            Zdcpnz_c(1:2,1) = Zdcpnz_c(1:2,1) + 0.25*abs(Xdcpnz_c(1,h+1))*abs(Ydcpnz_c(2,h+1))*[1;1].*exp(1i*((-angle(Xdcpnz_c(1,h+1))+angle(Ydcpnz_c(2,h+1)))*[1;-1]));
            Zdcpnz_c(1:2,1) = Zdcpnz_c(1:2,1) + 0.25*abs(Xdcpnz_c(1,h+1))*abs(Ydcpnz_c(3,h+1))*[1;1].*exp(1i*((-angle(Xdcpnz_c(1,h+1))+angle(Ydcpnz_c(3,h+1)))*[-1;1]));


            Zdcpnz_c(3,2*h+1) = Zdcpnz_c(3,2*h+1) + 0.5*Xdcpnz_c(2,h+1)*Ydcpnz_c(1,h+1)*exp(-1i*pi/2);


            Zdcpnz_c(1:2,1) = Zdcpnz_c(1:2,1) + 0.25*abs(Xdcpnz_c(2,h+1))*abs(Ydcpnz_c(1,h+1))*[1;1].*exp(1i*((-angle(Xdcpnz_c(2,h+1))+angle(Ydcpnz_c(1,h+1)))*[-1;1]));
            Zdcpnz_c(1:2,1) = Zdcpnz_c(1:2,1) + 0.25*abs(Xdcpnz_c(2,h+1))*abs(Ydcpnz_c(3,h+1))*[1;1].*exp(1i*((-angle(Xdcpnz_c(2,h+1))+angle(Ydcpnz_c(3,h+1)))*[1;-1]));
            
            Zdcpnz_c(1:2,1) = Zdcpnz_c(1:2,1) + 0.25*abs(Xdcpnz_c(3,h+1))*abs(Ydcpnz_c(1,h+1))*[1;1].*exp(1i*((-angle(Xdcpnz_c(3,h+1))+angle(Ydcpnz_c(1,h+1)))*[1;-1]));
            Zdcpnz_c(1:2,1) = Zdcpnz_c(1:2,1) + 0.25*abs(Xdcpnz_c(3,h+1))*abs(Ydcpnz_c(2,h+1))*[1;1].*exp(1i*((-angle(Xdcpnz_c(3,h+1))+angle(Ydcpnz_c(2,h+1)))*[-1;+1]));

            %%%%%%%%%%%%%%%%% POSITIVE (Ydc*Xp) %%%%%%%%%%%%%%%%%%%
            Zdcpnz_c(:,h+1) = Zdcpnz_c(:,h+1) + T312*Ydcpnz_c(:,1)*Xdcpnz_c(1,h+1); %[0 0 1; 1 0 0; 0 1 0]
            %%%%%%%%%%%%%%%%% POSITIVE (Xdc*Yp) %%%%%%%%%%%%%%%%%%%
            Zdcpnz_c(:,h+1) = Zdcpnz_c(:,h+1) + T312*Xdcpnz_c(:,1)*Ydcpnz_c(1,h+1);
            %%%%%%%%%%%%%%%%% NEGATIVE (Ydc*Xn) %%%%%%%%%%%%%%%%%%%
            Zdcpnz_c(:,h+1) = Zdcpnz_c(:,h+1) + T231*Ydcpnz_c(:,1)*Xdcpnz_c(2,h+1);
            %%%%%%%%%%%%%%%%% NEGATIVE (Xdc*Yn) %%%%%%%%%%%%%%%%%%%
            Zdcpnz_c(:,h+1) = Zdcpnz_c(:,h+1) + T231*Xdcpnz_c(:,1)*Ydcpnz_c(2,h+1);
            %%%%%%%%%%%%%%%%%%%%%%%%%%%%%%%%%%%%%%%%%%%%%%%%%%%%%%
            Zdcpnz_c(:,h+1) = Zdcpnz_c(:,h+1) + Ydcpnz_c(:,1)*Xdcpnz_c(3,h+1);
            %%%%%%%%%%%%%%%%%%%%%%%%%%%%%%%%%%%%%%%%%%%%%%%%%%%%%%
            Zdcpnz_c(:,h+1) = Zdcpnz_c(:,h+1) + Xdcpnz_c(:,1)*Ydcpnz_c(3,h+1);
            
%%%%%%%%%%%%%%%%%%%%%% h<=N ODD %%%%%%%%%%%%%%%%%%%%%%%%%%%%%%%%%%%%%%%%%
            if(mod(h,2)==1) 
                %%%%%%%%%%%%%%%%% D3p (3ph+) %%%%%%%%%%%%%%%%%%%%%%%

                %&%%%%%%%%%%%%%%%%%%%%%%%%%% PP + NN %%%%%%%%%%%%%%%%%%%%%%%%%%%
                for i = 1 : h - 1
                   Zdcpnz_c(1,h+1) = Zdcpnz_c(1,h+1) +    0.5*( real(Xdcpnz_c(2,i+1))*imag(Ydcpnz_c(2,h-i+1)) + imag(Xdcpnz_c(2,i+1))*real(Ydcpnz_c(2,h-i+1)) );
                   Zdcpnz_c(1,h+1) = Zdcpnz_c(1,h+1) + 1i*0.5*( -real(Xdcpnz_c(2,i+1))*real(Ydcpnz_c(2,h-i+1)) + imag(Xdcpnz_c(2,i+1))*imag(Ydcpnz_c(2,h-i+1)) );

                   Zdcpnz_c(2,h+1) = Zdcpnz_c(2,h+1) +    0.5*( real(Xdcpnz_c(1,i+1))*imag(Ydcpnz_c(1,h-i+1)) + imag(Xdcpnz_c(1,i+1))*real(Ydcpnz_c(1,h-i+1)) );
                   Zdcpnz_c(2,h+1) = Zdcpnz_c(2,h+1) + 1i*0.5*( -real(Xdcpnz_c(1,i+1))*real(Ydcpnz_c(1,h-i+1)) + imag(Xdcpnz_c(1,i+1))*imag(Ydcpnz_c(1,h-i+1)) );
                end

                for i = 1 : N - h

                    Zdcpnz_c(3,h+1) = Zdcpnz_c(3,h+1) -    imag(0.5*Xdcpnz_c(1:2,i+1)'*Ydcpnz_c(1:2,i+h+1)) -    imag(0.5*Ydcpnz_c(1:2,i+1)'*Xdcpnz_c(1:2,i+h+1));
                    Zdcpnz_c(3,h+1) = Zdcpnz_c(3,h+1) + 1i*real(0.5*Xdcpnz_c(1:2,i+1)'*Ydcpnz_c(1:2,i+h+1)) + 1i*real(0.5*Ydcpnz_c(1:2,i+1)'*Xdcpnz_c(1:2,i+h+1));

                end
                %&%%%%%%%%%%%%%%%%%%%%%%%%%% PP + NN %%%%%%%%%%%%%%%%%%%%%%%%%%%

                for k = 1 : (N + mod(N+1,2) - h)/2
                    i = 2*k-1;
                    j = i+h;

                    Zdcpnz_c(1,h+1) = Zdcpnz_c(1,h+1) + (0.5*(Xdcpnz_c(:,i+1)'*T132*T213*Ydcpnz_c(:,j+1))*exp(+1i*pi/2)) ...
                                                      + (0.5*(Xdcpnz_c(:,j+1)'*T213*T132*Ydcpnz_c(:,i+1))*exp(-1i*pi/2))';

                    Zdcpnz_c(2,h+1) = Zdcpnz_c(2,h+1) + (0.5*(Xdcpnz_c(:,i+1)'*T132*T321*Ydcpnz_c(:,j+1))*exp(+1i*pi/2)) ...
                                                      + (0.5*(Xdcpnz_c(:,j+1)'*T321*T132*Ydcpnz_c(:,i+1))*exp(-1i*pi/2))';

                    Zdcpnz_c(3,h+1) = Zdcpnz_c(3,h+1) + (0.5*Xdcpnz_c(3,i+1)'*Ydcpnz_c(3,j+1)*exp(1i*pi/2)) ...
                                                      - (0.5*Xdcpnz_c(3,j+1)'*Ydcpnz_c(3,i+1)*exp(1i*pi/2))';
                end

                for k = 1 : (N + mod(N,2) - h - 1)/2
                    i = 2*k;
                    j = i+h;
                    
                    Zdcpnz_c(1,h+1) = Zdcpnz_c(1,h+1) + (0.5*(Xdcpnz_c(:,i+1)'*T132*T213*Ydcpnz_c(:,j+1))*exp(+1i*pi/2)) ...
                                                      + (0.5*(Xdcpnz_c(:,j+1)'*T213*T132*Ydcpnz_c(:,i+1))*exp(-1i*pi/2))';

                    Zdcpnz_c(2,h+1) = Zdcpnz_c(2,h+1) + (0.5*(Xdcpnz_c(:,i+1)'*T132*T321*Ydcpnz_c(:,j+1))*exp(+1i*pi/2)) ...
                                                      + (0.5*(Xdcpnz_c(:,j+1)'*T321*T132*Ydcpnz_c(:,i+1))*exp(-1i*pi/2))';

                    Zdcpnz_c(3,h+1) = Zdcpnz_c(3,h+1) + (0.5*Xdcpnz_c(3,i+1)'*Ydcpnz_c(3,j+1)*exp(1i*pi/2)) ...
                                                      - (0.5*Xdcpnz_c(3,j+1)'*Ydcpnz_c(3,i+1)*exp(1i*pi/2))';
                end

                for k = (h-1)/2:-1:1
                    i = k;
                    j = h-i;  

                    Zdcpnz_c(3,h+1) = Zdcpnz_c(3,h+1) + 0.5*(real(Xdcpnz_c(:,i+1))'*T213*imag(Ydcpnz_c(:,j+1)) + imag(Xdcpnz_c(:,i+1))'*T213*real(Ydcpnz_c(:,j+1)) ...
                                                           + real(Xdcpnz_c(:,j+1))'*T213*imag(Ydcpnz_c(:,i+1)) + imag(Xdcpnz_c(:,j+1))'*T213*real(Ydcpnz_c(:,i+1)));
                                                                                       
                    Zdcpnz_c(3,h+1) = Zdcpnz_c(3,h+1) + 1i*0.5*(-real(Xdcpnz_c(:,i+1))'*T213*real(Ydcpnz_c(:,j+1)) + imag(Xdcpnz_c(:,i+1))'*T213*imag(Ydcpnz_c(:,j+1)) ...
                                                           - real(Xdcpnz_c(:,j+1))'*T213*real(Ydcpnz_c(:,i+1)) + imag(Xdcpnz_c(:,j+1))'*T213*imag(Ydcpnz_c(:,i+1)));

                    Zdcpnz_c(1,h+1) = Zdcpnz_c(1,h+1) + 0.5*(real(Xdcpnz_c([1,3],i+1))'*[0 1; 1 0]*imag(Ydcpnz_c([1,3],j+1)) + imag(Xdcpnz_c([1,3],i+1))'*[0 1; 1 0]*real(Ydcpnz_c([1,3],j+1)) ...
                                                           + real(Xdcpnz_c([1,3],j+1))'*[0 1; 1 0]*imag(Ydcpnz_c([1,3],i+1)) + imag(Xdcpnz_c([1,3],j+1))'*[0 1; 1 0]*real(Ydcpnz_c([1,3],i+1)) );

                    Zdcpnz_c(1,h+1) = Zdcpnz_c(1,h+1) + 1i*0.5*(-real(Xdcpnz_c([1,3],i+1))'*[0 1; 1 0]*real(Ydcpnz_c([1,3],j+1)) + imag(Xdcpnz_c([1,3],i+1))'*[0 1; 1 0]*imag(Ydcpnz_c([1,3],j+1)) ...
                                                              - real(Xdcpnz_c([1,3],j+1))'*[0 1; 1 0]*real(Ydcpnz_c([1,3],i+1)) + imag(Xdcpnz_c([1,3],j+1))'*[0 1; 1 0]*imag(Ydcpnz_c([1,3],i+1)) );

                    Zdcpnz_c(2,h+1) = Zdcpnz_c(2,h+1) + 0.5*(real(Xdcpnz_c([2,3],i+1))'*[0 1; 1 0]*imag(Ydcpnz_c([2,3],j+1)) + imag(Xdcpnz_c([2,3],i+1))'*[0 1; 1 0]*real(Ydcpnz_c([2,3],j+1)) ...
                                                           + real(Xdcpnz_c([2,3],j+1))'*[0 1; 1 0]*imag(Ydcpnz_c([2,3],i+1)) + imag(Xdcpnz_c([2,3],j+1))'*[0 1; 1 0]*real(Ydcpnz_c([2,3],i+1)) );

                    Zdcpnz_c(2,h+1) = Zdcpnz_c(2,h+1) + 1i*0.5*(-real(Xdcpnz_c([2,3],i+1))'*[0 1; 1 0]*real(Ydcpnz_c([2,3],j+1)) + imag(Xdcpnz_c([2,3],i+1))'*[0 1; 1 0]*imag(Ydcpnz_c([2,3],j+1)) ...
                                                              - real(Xdcpnz_c([2,3],j+1))'*[0 1; 1 0]*real(Ydcpnz_c([2,3],i+1)) + imag(Xdcpnz_c([2,3],j+1))'*[0 1; 1 0]*imag(Ydcpnz_c([2,3],i+1)) );

                end
%%%%%%%%%%%%%%%%%%%%%% h<=N EVEN %%%%%%%%%%%%%%%%%%%%%%%%%%%%%%%%%%%%%%%%%           
            else  

                Zdcpnz_c(3,h+1) = Zdcpnz_c(3,h+1) + 0.5*imag(Xdcpnz_c(3,h/2+1)*Ydcpnz_c(3,h/2+1))           -0.5*1i*real(Xdcpnz_c(3,h/2+1)*Ydcpnz_c(3,h/2+1));
                Zdcpnz_c(1,h+1) = Zdcpnz_c(1,h+1) + 0.5*real(Xdcpnz_c(:,h/2+1))'*T321*imag(Ydcpnz_c(:,h/2+1)) + 0.5*imag(Xdcpnz_c(:,h/2+1))'*T321*real(Ydcpnz_c(:,h/2+1));
                Zdcpnz_c(1,h+1) = Zdcpnz_c(1,h+1) - 0.5*1i*real(Xdcpnz_c(:,h/2+1))'*T321*real(Ydcpnz_c(:,h/2+1)) + 0.5*1i*imag(Xdcpnz_c(:,h/2+1))'*T321*imag(Ydcpnz_c(:,h/2+1));
                Zdcpnz_c(2,h+1) = Zdcpnz_c(2,h+1) + 0.5*real(Xdcpnz_c(:,h/2+1))'*T132*imag(Ydcpnz_c(:,h/2+1)) + 0.5*imag(Xdcpnz_c(:,h/2+1))'*T132*real(Ydcpnz_c(:,h/2+1));
                Zdcpnz_c(2,h+1) = Zdcpnz_c(2,h+1) - 0.5*1i*real(Xdcpnz_c(:,h/2+1))'*T132*real(Ydcpnz_c(:,h/2+1)) + 0.5*1i*imag(Xdcpnz_c(:,h/2+1))'*T132*imag(Ydcpnz_c(:,h/2+1));
                
                for k = 1:N-h
                    i = k;
                    j = h+i;

                    Zdcpnz_c(1,h+1) = Zdcpnz_c(1,h+1) + 0.5*( - real(Xdcpnz_c(:,i+1))'*T231*imag(Ydcpnz_c(:,j+1)) + imag(Xdcpnz_c(:,i+1))'*T231*real(Ydcpnz_c(:,j+1)) ...
                                                              + real(Xdcpnz_c(:,j+1))'*T312*imag(Ydcpnz_c(:,i+1)) - imag(Xdcpnz_c(:,j+1))'*T312*real(Ydcpnz_c(:,i+1)));

                    Zdcpnz_c(1,h+1) = Zdcpnz_c(1,h+1) + 0.5*1i*( + real(Xdcpnz_c(:,i+1))'*T231*real(Ydcpnz_c(:,j+1)) + imag(Xdcpnz_c(:,i+1))'*T231*imag(Ydcpnz_c(:,j+1)) ...
                                                                 + real(Xdcpnz_c(:,j+1))'*T312*real(Ydcpnz_c(:,i+1)) + imag(Xdcpnz_c(:,j+1))'*T312*imag(Ydcpnz_c(:,i+1)));

                    Zdcpnz_c(2,h+1) = Zdcpnz_c(2,h+1) + 0.5*( - real(Xdcpnz_c(:,i+1))'*T312*imag(Ydcpnz_c(:,j+1)) + imag(Xdcpnz_c(:,i+1))'*T312*real(Ydcpnz_c(:,j+1)) ...
                                                              + real(Xdcpnz_c(:,j+1))'*T231*imag(Ydcpnz_c(:,i+1)) - imag(Xdcpnz_c(:,j+1))'*T231*real(Ydcpnz_c(:,i+1)));

                    Zdcpnz_c(2,h+1) = Zdcpnz_c(2,h+1) + 1i*0.5*( + real(Xdcpnz_c(:,i+1))'*T312*real(Ydcpnz_c(:,j+1)) + imag(Xdcpnz_c(:,i+1))'*T312*imag(Ydcpnz_c(:,j+1)) ...
                                                              + real(Xdcpnz_c(:,j+1))'*T231*real(Ydcpnz_c(:,i+1)) + imag(Xdcpnz_c(:,j+1))'*T231*imag(Ydcpnz_c(:,i+1)));

                    Zdcpnz_c(3,h+1) = Zdcpnz_c(3,h+1) + 0.5*(-real(Xdcpnz_c(:,i+1))'*imag(Ydcpnz_c(:,j+1))+imag(Xdcpnz_c(:,i+1))'*real(Ydcpnz_c(:,j+1)) ...
                                                             +real(Xdcpnz_c(:,j+1))'*imag(Ydcpnz_c(:,i+1))-imag(Xdcpnz_c(:,j+1))'*real(Ydcpnz_c(:,i+1)));

                    Zdcpnz_c(3,h+1) = Zdcpnz_c(3,h+1) + 0.5*1i*(+real(Xdcpnz_c(:,i+1))'*real(Ydcpnz_c(:,j+1))+imag(Xdcpnz_c(:,i+1))'*imag(Ydcpnz_c(:,j+1)) ...
                                                             +real(Xdcpnz_c(:,j+1))'*real(Ydcpnz_c(:,i+1))+imag(Xdcpnz_c(:,j+1))'*imag(Ydcpnz_c(:,i+1)));

                end

                for k = h/2-1:-1:1
                    i = k;
                    j = h-i;   

                    Zdcpnz_c(3,h+1) = Zdcpnz_c(3,h+1) +    0.5*(+real(Xdcpnz_c(:,i+1))'*T213*imag(Ydcpnz_c(:,j+1)) + real(Xdcpnz_c(:,j+1))'*T213*imag(Ydcpnz_c(:,i+1)) + imag(Xdcpnz_c(:,i+1))'*T213*real(Ydcpnz_c(:,j+1)) + imag(Xdcpnz_c(:,j+1))'*T213*real(Ydcpnz_c(:,i+1)));

                    Zdcpnz_c(3,h+1) = Zdcpnz_c(3,h+1) + 1i*0.5*(-real(Xdcpnz_c(:,i+1))'*T213*real(Ydcpnz_c(:,j+1)) - real(Xdcpnz_c(:,j+1))'*T213*real(Ydcpnz_c(:,i+1)) + imag(Xdcpnz_c(:,i+1))'*T213*imag(Ydcpnz_c(:,j+1)) + imag(Xdcpnz_c(:,j+1))'*T213*imag(Ydcpnz_c(:,i+1)));

                    Zdcpnz_c(1,h+1) = Zdcpnz_c(1,h+1) + 0.5*( + real(Xdcpnz_c(:,i+1))'*T321*imag(Ydcpnz_c(:,j+1)) + imag(Xdcpnz_c(:,i+1))'*T321*real(Ydcpnz_c(:,j+1)) ...
                                                              + real(Xdcpnz_c(:,j+1))'*T321*imag(Ydcpnz_c(:,i+1)) + imag(Xdcpnz_c(:,j+1))'*T321*real(Ydcpnz_c(:,i+1)));


                    Zdcpnz_c(1,h+1) = Zdcpnz_c(1,h+1) + 0.5*1i*( - real(Xdcpnz_c(:,i+1))'*T321*real(Ydcpnz_c(:,j+1)) + imag(Xdcpnz_c(:,i+1))'*T321*imag(Ydcpnz_c(:,j+1)) ...
                                                                 - real(Xdcpnz_c(:,j+1))'*T321*real(Ydcpnz_c(:,i+1)) + imag(Xdcpnz_c(:,j+1))'*T321*imag(Ydcpnz_c(:,i+1)));
                    
                    Zdcpnz_c(2,h+1) = Zdcpnz_c(2,h+1) + 0.5*( + real(Xdcpnz_c(:,i+1))'*T132*imag(Ydcpnz_c(:,j+1)) + imag(Xdcpnz_c(:,i+1))'*T132*real(Ydcpnz_c(:,j+1)) ...
                                                              + real(Xdcpnz_c(:,j+1))'*T132*imag(Ydcpnz_c(:,i+1)) + imag(Xdcpnz_c(:,j+1))'*T132*real(Ydcpnz_c(:,i+1)));

                    Zdcpnz_c(2,h+1) = Zdcpnz_c(2,h+1) + 1i*0.5*( - real(Xdcpnz_c(:,i+1))'*T132*real(Ydcpnz_c(:,j+1)) + imag(Xdcpnz_c(:,i+1))'*T132*imag(Ydcpnz_c(:,j+1)) ...
                                                                 - real(Xdcpnz_c(:,j+1))'*T132*real(Ydcpnz_c(:,i+1)) + imag(Xdcpnz_c(:,j+1))'*T132*imag(Ydcpnz_c(:,i+1)));

                end
            end
%%%%%%%%%%%%%%%%%%%%%%%%%%%% h>N  %%%%%%%%%%%%%%%%%%%%%%%%%%%%%%%%%%%%%%%%% 
        else %h>N
            if(HrmDbl)
            
                %%%%%%%%%%%%%%%%%%%%%%%%%%% PP + NN %%%%%%%%%%%%%%%%%%%%%%%%%%%
                for i = h-N : N
                    Zdcpnz_c(1,h+1) = Zdcpnz_c(1,h+1) +    0.5*( real(Xdcpnz_c(2,i+1))*imag(Ydcpnz_c(2,h-i+1)) + imag(Xdcpnz_c(2,i+1))*real(Ydcpnz_c(2,h-i+1)) );
                    Zdcpnz_c(1,h+1) = Zdcpnz_c(1,h+1) + 1i*0.5*( -real(Xdcpnz_c(2,i+1))*real(Ydcpnz_c(2,h-i+1)) + imag(Xdcpnz_c(2,i+1))*imag(Ydcpnz_c(2,h-i+1)) );

                    Zdcpnz_c(2,h+1) = Zdcpnz_c(2,h+1) +    0.5*( real(Xdcpnz_c(1,i+1))*imag(Ydcpnz_c(1,h-i+1)) + imag(Xdcpnz_c(1,i+1))*real(Ydcpnz_c(1,h-i+1)) );
                    Zdcpnz_c(2,h+1) = Zdcpnz_c(2,h+1) + 1i*0.5*( -real(Xdcpnz_c(1,i+1))*real(Ydcpnz_c(1,h-i+1)) + imag(Xdcpnz_c(1,i+1))*imag(Ydcpnz_c(1,h-i+1)) );
                end
                %%%%%%%%%%%%%%%%%%%%%%%%%%% PP + NN %%%%%%%%%%%%%%%%%%%%%%%%%%%

                if(mod(h,2)==1) %%%%%%%%%%% h>N ODD %%%%%%%%%%%%%%%%%%%

                    for k = (h-1)/2:-1:h-N
                        i = k;  %%%
                        j = h-i;

                        Zdcpnz_c(1,h+1) = Zdcpnz_c(1,h+1) + 0.5*( + real(Xdcpnz_c([1,3],i+1))'*imag(Ydcpnz_c([3,1],j+1)) + imag(Xdcpnz_c([1,3],i+1))'*real(Ydcpnz_c([3,1],j+1)) ...
                                                                  + real(Xdcpnz_c([1,3],j+1))'*imag(Ydcpnz_c([3,1],i+1)) + imag(Xdcpnz_c([1,3],j+1))'*real(Ydcpnz_c([3,1],i+1)));

                        Zdcpnz_c(1,h+1) = Zdcpnz_c(1,h+1) + 1i*0.5*( - real(Xdcpnz_c([1,3],i+1))'*real(Ydcpnz_c([3,1],j+1)) + imag(Xdcpnz_c([1,3],i+1))'*imag(Ydcpnz_c([3,1],j+1)) ...
                                                                     - real(Xdcpnz_c([1,3],j+1))'*real(Ydcpnz_c([3,1],i+1)) + imag(Xdcpnz_c([1,3],j+1))'*imag(Ydcpnz_c([3,1],i+1)));

                        Zdcpnz_c(2,h+1) = Zdcpnz_c(2,h+1) + 0.5*( + real(Xdcpnz_c([2,3],i+1))'*imag(Ydcpnz_c([3,2],j+1)) + imag(Xdcpnz_c([2,3],i+1))'*real(Ydcpnz_c([3,2],j+1)) ...
                                                                  + real(Xdcpnz_c([2,3],j+1))'*imag(Ydcpnz_c([3,2],i+1)) + imag(Xdcpnz_c([2,3],j+1))'*real(Ydcpnz_c([3,2],i+1)));

                        Zdcpnz_c(2,h+1) = Zdcpnz_c(2,h+1) + 1i*0.5*( - real(Xdcpnz_c([2,3],i+1))'*real(Ydcpnz_c([3,2],j+1)) + imag(Xdcpnz_c([2,3],i+1))'*imag(Ydcpnz_c([3,2],j+1)) ...
                                                                     - real(Xdcpnz_c([2,3],j+1))'*real(Ydcpnz_c([3,2],i+1)) + imag(Xdcpnz_c([2,3],j+1))'*imag(Ydcpnz_c([3,2],i+1)));

                        Zdcpnz_c(3,h+1) = Zdcpnz_c(3,h+1) +    0.5*(+real(Xdcpnz_c(:,i+1))'*T213*imag(Ydcpnz_c(:,j+1)) + real(Xdcpnz_c(:,j+1))'*T213*imag(Ydcpnz_c(:,i+1)) + imag(Xdcpnz_c(:,i+1))'*T213*real(Ydcpnz_c(:,j+1)) + imag(Xdcpnz_c(:,j+1))'*T213*real(Ydcpnz_c(:,i+1)));
                        Zdcpnz_c(3,h+1) = Zdcpnz_c(3,h+1) + 1i*0.5*(-real(Xdcpnz_c(:,i+1))'*T213*real(Ydcpnz_c(:,j+1)) - real(Xdcpnz_c(:,j+1))'*T213*real(Ydcpnz_c(:,i+1)) + imag(Xdcpnz_c(:,i+1))'*T213*imag(Ydcpnz_c(:,j+1)) + imag(Xdcpnz_c(:,j+1))'*T213*imag(Ydcpnz_c(:,i+1)));

                    end

                else %%%%%%%%%%% h>N EVEN %%%%%%%%%%%%%%%%%%%

                    Zdcpnz_c(1,h+1) = 0.5*real(Xdcpnz_c(:,h/2+1))'*T321*imag(Ydcpnz_c(:,h/2+1)) + 0.5*imag(Xdcpnz_c(:,h/2+1))'*T321*real(Ydcpnz_c(:,h/2+1)) - 0.5*1i*real(Xdcpnz_c(:,h/2+1))'*T321*real(Ydcpnz_c(:,h/2+1)) + 0.5*1i*imag(Xdcpnz_c(:,h/2+1))'*T321*imag(Ydcpnz_c(:,h/2+1));
                    Zdcpnz_c(2,h+1) = 0.5*real(Xdcpnz_c(:,h/2+1))'*T132*imag(Ydcpnz_c(:,h/2+1)) + 0.5*imag(Xdcpnz_c(:,h/2+1))'*T132*real(Ydcpnz_c(:,h/2+1))- 0.5*1i*real(Xdcpnz_c(:,h/2+1))'*T132*real(Ydcpnz_c(:,h/2+1)) + 0.5*1i*imag(Xdcpnz_c(:,h/2+1))'*T132*imag(Ydcpnz_c(:,h/2+1));
                    Zdcpnz_c(3,h+1) = Zdcpnz_c(3,h+1) + 0.5*imag(Xdcpnz_c(3,h/2+1)*Ydcpnz_c(3,h/2+1)) - 1i*0.5*real(Xdcpnz_c(3,h/2+1)*Ydcpnz_c(3,h/2+1));


                    for i = (h+2)/2:N
                        j = h-i;

                        Zdcpnz_c(1,h+1) = Zdcpnz_c(1,h+1) + 0.5*( + real(Xdcpnz_c(:,i+1))'*T321*imag(Ydcpnz_c(:,j+1)) + imag(Xdcpnz_c(:,i+1))'*T321*real(Ydcpnz_c(:,j+1)) ...
                                                                  + real(Xdcpnz_c(:,j+1))'*T321*imag(Ydcpnz_c(:,i+1)) + imag(Xdcpnz_c(:,j+1))'*T321*real(Ydcpnz_c(:,i+1)));
    
                        Zdcpnz_c(1,h+1) = Zdcpnz_c(1,h+1) + 0.5*1i*( - real(Xdcpnz_c(:,i+1))'*T321*real(Ydcpnz_c(:,j+1)) + imag(Xdcpnz_c(:,i+1))'*T321*imag(Ydcpnz_c(:,j+1)) ...
                                                                     - real(Xdcpnz_c(:,j+1))'*T321*real(Ydcpnz_c(:,i+1)) + imag(Xdcpnz_c(:,j+1))'*T321*imag(Ydcpnz_c(:,i+1)));

                        Zdcpnz_c(2,h+1) = Zdcpnz_c(2,h+1) + 0.5*( + real(Xdcpnz_c(:,i+1))'*T132*imag(Ydcpnz_c(:,j+1)) + imag(Xdcpnz_c(:,i+1))'*T132*real(Ydcpnz_c(:,j+1)) ...
                                                                  + real(Xdcpnz_c(:,j+1))'*T132*imag(Ydcpnz_c(:,i+1)) + imag(Xdcpnz_c(:,j+1))'*T132*real(Ydcpnz_c(:,i+1)));
    
                        Zdcpnz_c(2,h+1) = Zdcpnz_c(2,h+1) + 0.5*1i*( - real(Xdcpnz_c(:,i+1))'*T132*real(Ydcpnz_c(:,j+1)) + imag(Xdcpnz_c(:,i+1))'*T132*imag(Ydcpnz_c(:,j+1)) ...
                                                                     - real(Xdcpnz_c(:,j+1))'*T132*real(Ydcpnz_c(:,i+1)) + imag(Xdcpnz_c(:,j+1))'*T132*imag(Ydcpnz_c(:,i+1)));

                        Zdcpnz_c(3,h+1) = Zdcpnz_c(3,h+1) +    0.5*(+real(Xdcpnz_c(:,i+1))'*T213*imag(Ydcpnz_c(:,j+1)) + real(Xdcpnz_c(:,j+1))'*T213*imag(Ydcpnz_c(:,i+1)) + imag(Xdcpnz_c(:,i+1))'*T213*real(Ydcpnz_c(:,j+1)) + imag(Xdcpnz_c(:,j+1))'*T213*real(Ydcpnz_c(:,i+1)));
                        Zdcpnz_c(3,h+1) = Zdcpnz_c(3,h+1) + 1i*0.5*(-real(Xdcpnz_c(:,i+1))'*T213*real(Ydcpnz_c(:,j+1)) - real(Xdcpnz_c(:,j+1))'*T213*real(Ydcpnz_c(:,i+1)) + imag(Xdcpnz_c(:,i+1))'*T213*imag(Ydcpnz_c(:,j+1)) + imag(Xdcpnz_c(:,j+1))'*T213*imag(Ydcpnz_c(:,i+1)));

                    end
                end
            end
        end  
    end
    

end

== matlab function DQN_Lib (conflicted copy 2023-11-25 155310)/DQn->ABC6 ==
  data: Xdcpnz_c input; tho input; Xabc output; N parameter
%function abc = Mult(Z0,Zdp,Zqp,Zdn,Zqn,Zdz,Zqz,th, N)
function Xabc = dqn2abc(Xdcpnz_c,tho,N)

    persistent Sas;
    persistent Ssa;

    if(isempty(Sas)) 
        a = -0.5+0.866i;
        a2 = -0.5-0.866i;
        Sas = [1,a,a2;1,a2,a;1,1,1]/3;
        Ssa = eye(3)/(Sas);
    end

    Xabc = zeros(3,1);

    for i = 1 : N+1
    
    
        if(i>1)
            h = i-1;
    
            th = h*tho;
        
            mag_p = abs(Xdcpnz_c(1,i));
            ang_p = angle(Xdcpnz_c(1,i));
            mag_n = abs(Xdcpnz_c(2,i));
            ang_n = angle(Xdcpnz_c(2,i));
            mag_z = abs(Xdcpnz_c(3,i));
            ang_z = angle(Xdcpnz_c(3,i));
            
            abc3p = mag_p*[sin(th+ang_p) ; sin(th+ang_p-2*pi/3) ; sin(th+ang_p+2*pi/3) ];
            abc3n = mag_n*[sin(th+ang_n) ; sin(th+ang_n+2*pi/3) ; sin(th+ang_n-2*pi/3) ];
            abc3z = mag_z*[sin(th+ang_z) ; sin(th+ang_z)        ; sin(th+ang_z)  ];
        
            Xabc = Xabc + abc3p+abc3n+abc3z;
        else
            Xabc = Xabc + real(Ssa*(Xdcpnz_c(:,1)));
        
        end
    
        
    end

end

== matlab function DQN_Lib (conflicted copy 2023-11-25 155310)/Der_DQNc_Mat ==
  data: Xpnz input; N parameter; Zpnz output; w parameter; EMT parameter; Ts parameter; sw_soft parameter
function Zpnz    = fMultDQNc(Xpnz, N, w, EMT, Ts, sw_soft)
    Zpnz = complex(zeros(3,N+1));

    sX = size(Xpnz,2);
    Xpnz = [Xpnz zeros(3,N+1-sX)];

    persistent Xpnz_old;
    persistent firstStep;

    if(isempty(Xpnz_old)) 
        Xpnz_old = complex(zeros(3,N+1));
        firstStep = 0;

    end


        for h = 2 : N + 1
            wn = (h-1)*w;
            if(EMT)
                if(sw_soft==1 && firstStep == 0)
                    Xpnz_old(:,h) = Xpnz(:,h);
                else
                    Zpnz(:,h) = (Xpnz(:,h)-Xpnz_old(:,h))/Ts;
                    Xpnz_old(:,h) = Xpnz(:,h);
                end

            end

            Zpnz(:,h) = Zpnz(:,h) + 1i*wn*Xpnz(:,h);

            firstStep = 1;
        end
    
end

== matlab function DQN_Lib (conflicted copy 2023-11-25 155310)/BACKUP/Int_DQNc_Mat ==
  settings: updateMethod=DISCRETE
  data: Xpnz input; N parameter; dt parameter; w parameter; InitInt parameter; Zpnz output
function Zpnz    = Int_DQN_Mat(Xpnz, N, dt, w, InitInt)

    nrSig = 1;

    Zpnz = complex(zeros(3,N+1));

    persistent Zpnz_old;
    persistent Xpnz_old;


        dt2 = dt/2;
        
    if(isempty(Zpnz_old)) 
    
        a = -0.5+0.866i;
        a2 = -0.5-0.866i;
        Sas = [1,a,a2;1,a2,a;1,1,1]/3;
        
        Zpnz_old = complex(zeros(3,N+1));
        Xpnz_old = complex(zeros(3,N+1));
        
        if(~isempty(InitInt))
        Zpnz_old(:,1) = Sas * InitInt;
        
        end
            
    end
       
    
    for k = 1 : nrSig
    
        Zpnz(:,1) = dt2*(Xpnz(:,1)+Xpnz_old(:,1)) + Zpnz_old(:,1);

        Xpnz_old(:,1) = Xpnz(:,1);
        Zpnz_old(:,1) = Zpnz(:,1);


        if(N>0)

            for i = 1 : N
                wn =  i * w; 

                wndt2 = wn*dt2;
                A = 1/(1+(dt2*wn)^2);

                %%% POS %%%
                K1 = dt*real(Xpnz(1,i+1)) + real(Zpnz_old(1,i+1))      + imag(Zpnz_old(1,i+1))*wndt2;
                K2 = dt*imag(Xpnz(1,i+1)) -real(Zpnz_old(1,i+1))*wndt2 + imag(Zpnz_old(1,i+1));

                % Zdp(i) = (A)*( real(Xpnz(1,i+1))+imag(Zpnz_old(1,i+1))*wndt2/dt2 + real(Zpnz_old(1,i+1))*(1-wndt2^2)/2/dt2 + wndt2*imag(Xpnz(1,i+1)) );
                % Zqp(i) = (A)*( imag(Xpnz(1,i+1))-real(Zpnz_old(1,i+1))*wndt2/dt2 + imag(Zpnz_old(1,i+1))*(1-wndt2^2)/2/dt2 - wndt2*real(Xpnz(1,i+1)) );

                Zpnz(1,i+1) = A*( ( K1 + wndt2*K2) + 1i*( K2 - wndt2*K1) );

                %%% NEG %%%
                K1 = dt2*(2*real(Xpnz(2,i+1))+imag(Zpnz_old(2,i+1))*wn) + real(Zpnz_old(2,i+1));
                K2 = dt2*(2*imag(Xpnz(2,i+1))-real(Zpnz_old(2,i+1))*wn) + imag(Zpnz_old(2,i+1));

                Zpnz(2,i+1) = A*( K1 + wndt2*K2) + 1i*A*( K2 - wndt2*K1);

                %%% ZERO %%%
                K1 = dt2*(2*real(Xpnz(3,i+1))+imag(Zpnz_old(3,i+1))*wn) + real(Zpnz_old(3,i+1));
                K2 = dt2*(2*imag(Xpnz(3,i+1))-real(Zpnz_old(3,i+1))*wn) + imag(Zpnz_old(3,i+1));

                Zpnz(3,i+1) = A*( K1 + wndt2*K2) + 1i*A*( K2 - wndt2*K1);
                Zpnz_old(:,i+1) = Zpnz(:,i+1);


            end

        end

    end
end
